simulink model "LQ_controller_acsus_final_with_LQ_controller_final"  (R2021a)
settings: Solver=VariableStepAuto  StartTime=0.0  StopTime=8  RelTol=1e-3
undefined symbols (not defined in the file): Cs, Cus, Ks, Kus, Ms, Mus
libraries: simulink x1
settings Model: Creator=rlsot  LastModifiedBy=rlsot

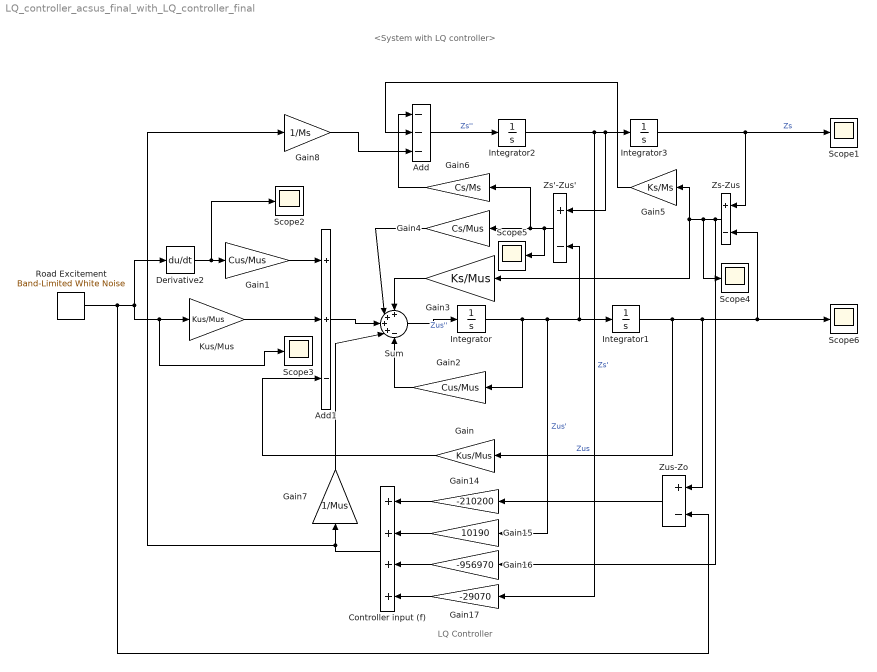
== system LQ_controller_acsus_final_with_LQ_controller_final ==
  note: LQ Controller
  note: <System with LQ controller>
  Add : Sum  Inputs=---
  Add1 : Sum  Inputs=++-
  Controller input (f) : Sum  Inputs=++++
  Derivative2 : Derivative
  Gain : Gain  Gain=Kus/Mus
  Gain1 : Gain  Gain=Cus/Mus
  Gain14 : Gain  Gain=-210200
  Gain15 : Gain  Gain=10190
  Gain16 : Gain  Gain=-956970
  Gain17 : Gain  Gain=-29070
  Gain2 : Gain  Gain=Cus/Mus
  Gain3 : Gain  Gain=Ks/Mus
  Gain4 : Gain  Gain=Cs/Mus
  Gain5 : Gain  Gain=Ks/Ms
  Gain6 : Gain  Gain=Cs/Ms
  Gain7 : Gain  Gain=1/Mus
  Gain8 : Gain  Gain=1/Ms
  Integrator{,1..3} (4 alike) : Integrator
  Kus/Mus : Gain  Gain=Kus/Mus
  Road Excitement : simulink/Sources/Band-Limited White Noise  Cov=[0.001]  Ts=0.01  seed=[23341]
  Scope{1..6} (6 alike) : Scope
  Sum : Sum  Inputs=++++-
  Zs'-Zus' : Sum  Inputs=+-
  Zs-Zus : Sum  Inputs=+-
  Zus-Zo : Sum  Inputs=+-
  wires:
  Zs'-Zus'/1 -> Scope5/1, Gain6/1, Gain4/1
  Gain6/1 -> Add/1
  Gain5/1 -> Add/2
  Sum/1 -> Integrator/1  "Zus''"
  Integrator3/1 -> Zs-Zus/1, Scope1/1  "Zs"
  Zs-Zus/1 -> Gain16/1, Scope4/1, Gain5/1, Gain3/1
  Add/1 -> Integrator2/1  "Zs''"
  Integrator1/1 -> Scope6/1, Zs-Zus/2, Zus-Zo/1, Gain/1  "Zus"
  Integrator2/1 -> Gain17/1, Zs'-Zus'/1, Integrator3/1  "Zs'"
  Kus/Mus/1 -> Add1/2
  Gain3/1 -> Sum/1
  Gain4/1 -> Sum/2
  Derivative2/1 -> Scope2/1, Gain1/1
  Integrator/1 -> Gain15/1, Zs'-Zus'/2, Integrator1/1, Gain2/1  "Zus'"
  Gain/1 -> Add1/3
  Gain1/1 -> Add1/1
  Road Excitement/1 -> Zus-Zo/2, Derivative2/1, Scope3/1, Kus/Mus/1
  Add1/1 -> Sum/3
  Gain2/1 -> Sum/5
  Zus-Zo/1 -> Gain14/1
  Gain14/1 -> Controller input (f)/1
  Gain15/1 -> Controller input (f)/2
  Gain16/1 -> Controller input (f)/3
  Gain17/1 -> Controller input (f)/4
  Controller input (f)/1 -> Gain8/1, Gain7/1
  Gain7/1 -> Sum/4
  Gain8/1 -> Add/3
